simulink model "PID_Estimator_Simulink_J2"  (R2017b)
settings: Solver=VariableStepAuto  StartTime=0.0  StopTime=90000  RelTol=1e-3
InitFcn:
  | load('Sim_Truth_SecondOrder_Corrected5.mat')
  | 
  | load('OCV_table.mat')
values from neighbouring files (symbols this model uses):
  A1 = A(1,1)    [PID_Code.m]
  A2 = A(2,2)    [PID_Code.m]
  B1 = B(1,1)    [PID_Code.m]
  B2 = B(2,1)    [PID_Code.m]
  C2 = C(1,2)    [PID_Code.m]
  D = -R0    (= -0.1)    [PID_Code.m]
  Vocv0 = 3.435    [PID_Code.m]
libraries: dspsrcs4 x3, simulink x1
settings Model: Creator=Indiana  LastModifiedBy=Indiana
settings SFSimCC: SimUseLocalCustomCode=on
settings RTWCC: RTWUseLocalCustomCode=on

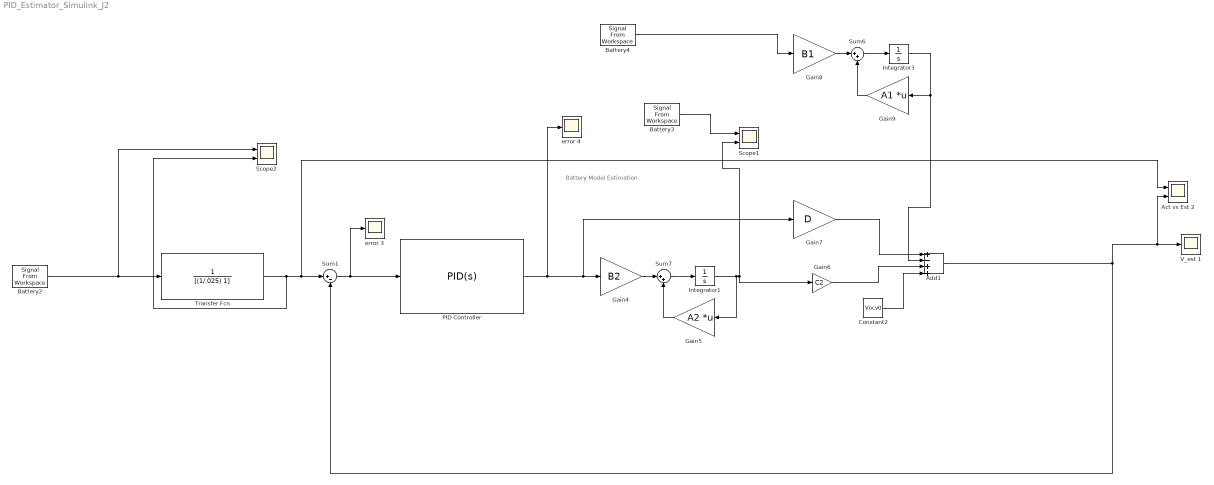
== system PID_Estimator_Simulink_J2 ==
  note: Battery Model Estimation
  Act vs Est 2 : Scope  NumInputPorts=2
  Add1 : Sum  Inputs=+-++
  Battery2 : dspsrcs4/Signal From Workspace  X=V  Ts=1  nsamps=1  OutputAfterFinalValue=Setting to zero  ignoreOrWarnInputAndFrameLengths=off  OutputFrames=off
  Battery3 : dspsrcs4/Signal From Workspace  X=SOC_act  Ts=1  nsamps=1  OutputAfterFinalValue=Setting to zero  ignoreOrWarnInputAndFrameLengths=off  OutputFrames=off
  Battery4 : dspsrcs4/Signal From Workspace  X=I  Ts=1  nsamps=1  OutputAfterFinalValue=Setting to zero  ignoreOrWarnInputAndFrameLengths=off  OutputFrames=off
  Constant2 : Constant  Value=Vocv0
  Gain4 : Gain  Gain=B2
  Gain5 : Gain  Gain=A2  Multiplication=Matrix(K*u)
  Gain6 : Gain  Gain=C2
  Gain7 : Gain  Gain=D
  Gain8 : Gain  Gain=B1
  Gain9 : Gain  Gain=A1  Multiplication=Matrix(K*u)
  Integrator1 : Integrator  InitialCondition=[.98]
  Integrator3 : Integrator  InitialCondition=[0]
  PID Controller : simulink/Continuous/PID Controller  Controller=PID  TimeDomain=Continuous-time  SampleTime=-1  IntegratorMethod=Forward Euler  FilterMethod=Forward Euler  Form=Parallel  UseFilter=on  ControllerParametersSource=internal  P=15  I=0  D=0  N=100  InitialConditionSource=internal  InitialConditionForIntegrator=0  InitialConditionForFilter=0  ExternalReset=none  LimitOutput=off  UpperSaturationLimit=inf  LowerSaturationLimit=-inf  LinearizeAsGain=on  AntiWindupMode=none  Kb=1  TrackingMode=off  Kt=1  PParamMin=[]  PParamMax=[]  IParamMin=[]  IParamMax=[]  DParamMin=[]  DParamMax=[]  NParamMin=[]  NParamMax=[]  KbParamMin=[]  KbParamMax=[]  KtParamMin=[]  KtParamMax=[]  POutMin=[]  POutMax=[]  IOutMin=[]  IOutMax=[]  DOutMin=[]  DOutMax=[]  NOutMin=[]  NOutMax=[]  KbOutMin=[]  KbOutMax=[]  KtOutMin=[]  KtOutMax=[]  IntegratorOutMin=[]  IntegratorOutMax=[]  FilterOutMin=[]  FilterOutMax=[]  SumOutMin=[]  SumOutMax=[]  SumI1OutMin=[]  SumI1OutMax=[]  SumI2OutMin=[]  SumI2OutMax=[]  SumI3OutMin=[]  SumI3OutMax=[]  SumDOutMin=[]  SumDOutMax=[]  SaturationOutMin=[]  SaturationOutMax=[]  IntegratorContinuousStateAttributes=''  IntegratorStateMustResolveToSignalObject=off  IntegratorRTWStateStorageClass=Auto  FilterContinuousStateAttributes=''  FilterStateMustResolveToSignalObject=off  FilterRTWStateStorageClass=Auto  DifferentiatorICPrevScaledInput=0  DifferentiatorOutMin=[]  DifferentiatorOutMax=[]  InitialConditionSetting=State (most efficient)  FilterDiffOutCoefMin=[]  FilterDiffOutCoefMax=[]  SumDenOutMin=[]  SumDenOutMax=[]  SumNumOutMin=[]  SumNumOutMax=[]  ReciprocalOutMin=[]  ReciprocalOutMax=[]  DivideOutMin=[]  DivideOutMax=[]  TunerSelectOption=Transfer Function Based (PID Tuner App)
  Scope1 : Scope  NumInputPorts=2
  Scope2 : Scope  NumInputPorts=2
  Sum1 : Sum  Inputs=|+-
  Sum6 : Sum  Inputs=|++
  Sum7 : Sum  Inputs=|++
  Transfer Fcn : TransferFcn  Denominator=[(1/.025) 1]
  V_est 1 : Scope
  error 3 : Scope
  error 4 : Scope
  wires:
  Gain4/1 -> Sum7/1
  Gain5/1 -> Sum7/2
  Sum7/1 -> Integrator1/1
  PID Controller/1 -> Gain7/1, Gain4/1, error 4/1
  Sum1/1 -> error 3/1, PID Controller/1
  Add1/1 -> V_est 1/1, Act vs Est 2/2, Sum1/2
  Battery3/1 -> Scope1/1
  Integrator1/1 -> Gain6/1, Scope1/2, Gain5/1
  Gain7/1 -> Add1/1
  Battery2/1 -> Transfer Fcn/1, Scope2/1
  Transfer Fcn/1 -> Scope2/2, Act vs Est 2/1, Sum1/1
  Gain9/1 -> Sum6/2
  Sum6/1 -> Integrator3/1
  Integrator3/1 -> Add1/2, Gain9/1
  Gain8/1 -> Sum6/1
  Battery4/1 -> Gain8/1
  Gain6/1 -> Add1/3
  Constant2/1 -> Add1/4
